simulink model "robot_lab"  (R2024b)
settings: Solver=FixedStepAuto  StartTime=0.0  StopTime=total_time  FixedStep=1e-2  RelTol=1e-3
values from neighbouring files (symbols this model uses):
  d_nom = 0.165    [MAIN_ROBOT.m]
  mode = 2    [MAIN_ROBOT.m]
  omega_L = (2*v - d_nom*w) ./ (2*r_nom)    [MAIN_ROBOT.m]
  omega_max = 10    [MAIN_ROBOT.m]
  omega_R = (2*v + d_nom*w) ./ (2*r_nom)    [MAIN_ROBOT.m]
  omega_trj = 2*pi    (= 6.28318530718)    [MAIN_ROBOT.m]
  R = 0.4    [MAIN_ROBOT.m]
  r_nom = 0.03    [MAIN_ROBOT.m]
  Ta = 1    [MAIN_ROBOT.m]
  Tc = 30    [MAIN_ROBOT.m]
  total_time = 35    [MAIN_ROBOT.m]
  Ts = 0.04    [MAIN_ROBOT.m]
undefined symbols (not defined in the file or in its folder): X, Y
libraries: robotlib x8, dspsigops x1
settings Model: SimulationMode=external  Creator=leontecosm  LastModifiedBy=leontecosm
settings OptimizationCC: DefaultParameterBehavior=Inlined  EnhancedBackFolding=on  PassReuseOutputArgsAs=Individual arguments  ZeroExternalMemoryAtStartup=off  ZeroInternalMemoryAtStartup=off  MaxStackSize=64  OptimizeBlockOrder=speed  DifferentSizesBufferReuse=on  OptimizationCustomize=off  EfficientTunableParamExpr=on
settings DebuggingCC: ParameterTunabilityLossMsg=error
settings HardwareCC: ProdBitPerPointer=32  ProdBitPerSizeT=32  ProdBitPerPtrDiffT=32  ProdLargestAtomicFloat=None  ProdIntDivRoundTo=Undefined  ProdEndianess=Unspecified  ProdWordSize=32  ProdHWDeviceType=Generic->Unspecified (assume 32-bit Generic)
settings SFSimCC: MATLABDynamicMemAlloc=off
settings RTWCC: Description=Embedded Coder  SystemTargetFile=ert.tlc  HardwareBoard=Robot Operating System (ROS)  TLCOptions="-aInlineSetEventsForThisBaseRateFcn=TLC_FALSE -aSuppressMultiTaskScheduler=TLC_FALSE  -aRateBasedStepFcn=0"  TemplateMakefile=ert_default_tmf  Toolchain=Catkin  TargetLang=C++
settings CodeAppCC: ForceParamTrailComments=on  IgnoreCustomStorageClasses=off  OperatorAnnotations=on  SimulinkDataObjDesc=on  SFDataObjDesc=on  InsertBlockDesc=on

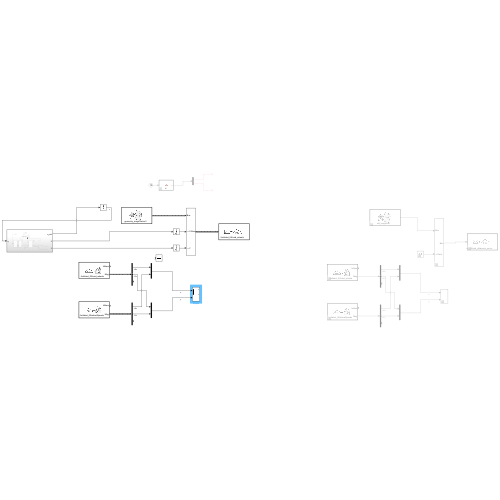
[thumbnail: Simulink's stored preview of the top-level diagram]
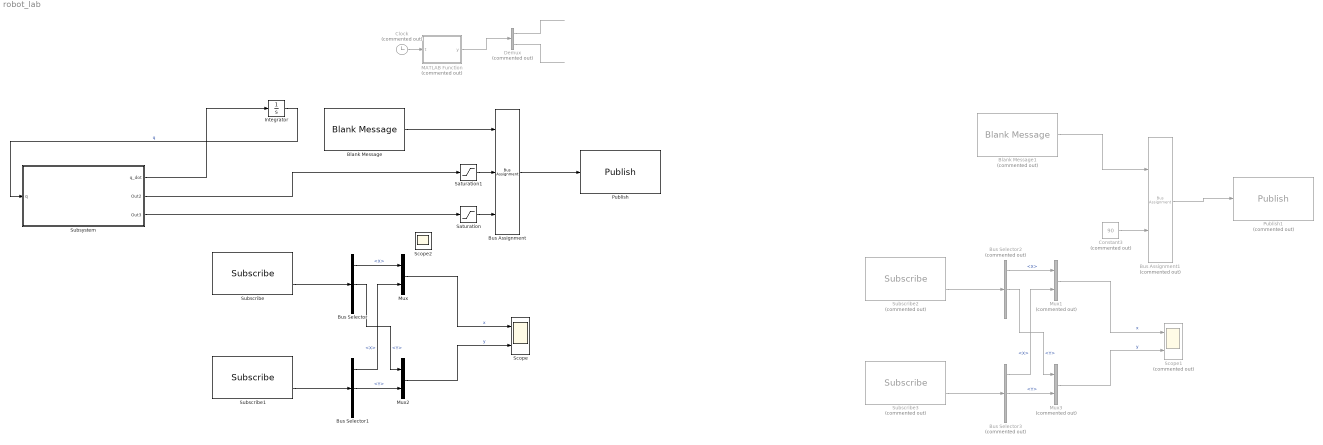
== system robot_lab ==
  Blank Message : robotlib/Blank Message  messageClass=Message  entityType=geometry_msgs/Vector3  messageType=geometry_msgs/Vector3  SampleTime=1e-2  legacyBusStruct=off
  Blank Message1 : robotlib/Blank Message  Commented=on  messageClass=Message  entityType=std_msgs/Int8  messageType=std_msgs/Int8  SampleTime=1e-1  legacyBusStruct=off
  Bus Assignment : BusAssignment  AssignedSignals=X,Y
  Bus Assignment1 : BusAssignment  Commented=on  AssignedSignals=Data
  Bus Selector : BusSelector  OutputSignals=X,Y,Z
  Bus Selector1 : BusSelector  OutputSignals=X,Y,Z
  Bus Selector2 : BusSelector  Commented=on  OutputSignals=X,Y,Z
  Bus Selector3 : BusSelector  Commented=on  OutputSignals=X,Y,Z
  Clock : Clock  Commented=on
      settings: Decimation=1/Ts
  Constant3 : Constant  Commented=on  Value=90  OutDataTypeStr=int8
  Demux : Demux  Commented=on  Outputs=2
  Integrator : Integrator  InitialCondition=[0,0,pi/3]'
  MATLAB Function : MATLAB Function  Commented=on  TreatAsAtomicUnit=on
  Mux : Mux  Inputs=2
  Mux1 : Mux  Commented=on  Inputs=2
  Mux2 : Mux  Inputs=2
  Mux3 : Mux  Commented=on  Inputs=2
  Publish : robotlib/Publish  topicSource=Select from ROS network  topic=/turtlebot_05/cmd_wheels  messageType=geometry_msgs/Vector3  legacyBusStruct=off  messageQueueLength=1
  Publish1 : robotlib/Publish  Commented=on  topicSource=Select from ROS network  topic=/turtlebot_05/cmd_ultrasonic_servo  messageType=std_msgs/Int8  legacyBusStruct=off  messageQueueLength=1
  Saturation : Saturate  UpperLimit=omega_max  LowerLimit=-omega_max
  Saturation1 : Saturate  UpperLimit=omega_max  LowerLimit=-omega_max
  Scope : Scope  NumInputPorts=2
  Scope1 : Scope  Commented=on  NumInputPorts=2
  Scope2 : Scope
  Subscribe : robotlib/Subscribe  topicSource=Select from ROS network  topic=/turtlebot_05/cmd_wheels  messageType=geometry_msgs/Vector3  SampleTime=1e-2  legacyBusStruct=off  messageQueueLength=1
  Subscribe1 : robotlib/Subscribe  topicSource=Select from ROS network  topic=/turtlebot_05/wheelSpeeds  messageType=geometry_msgs/Vector3  SampleTime=1e-2  legacyBusStruct=off  messageQueueLength=1
  Subscribe2 : robotlib/Subscribe  Commented=on  topicSource=Select from ROS network  topic=/turtlebot_05/cmd_wheels  messageType=geometry_msgs/Vector3  SampleTime=-1  legacyBusStruct=off  messageQueueLength=1
  Subscribe3 : robotlib/Subscribe  Commented=on  topicSource=Select from ROS network  topic=/turtlebot_05/wheelSpeeds  messageType=geometry_msgs/Vector3  SampleTime=-1  legacyBusStruct=off  messageQueueLength=1
  Subsystem : Subsystem
  wires:
  Blank Message/1 -> Bus Assignment/1
  Bus Assignment/1 -> Publish/1
  Saturation/1 -> Bus Assignment/3
  Saturation1/1 -> Bus Assignment/2
  Subscribe/2 -> Bus Selector/1
  Subscribe1/2 -> Bus Selector1/1
  Bus Selector/1 -> Mux/1  "<X>"
  Bus Selector1/1 -> Mux/2  "<X>"
  Bus Selector/2 -> Mux2/1  "<Y>"
  Bus Selector1/2 -> Mux2/2  "<Y>"
  Mux/1 -> Scope/1  "x"
  Mux2/1 -> Scope/2  "y"
  Mux3/1 -> Scope1/2  "y"
  Mux1/1 -> Scope1/1  "x"
  Bus Selector3/2 -> Mux3/2  "<Y>"
  Bus Selector2/2 -> Mux3/1  "<Y>"
  Bus Selector3/1 -> Mux1/2  "<X>"
  Bus Selector2/1 -> Mux1/1  "<X>"
  Subscribe3/2 -> Bus Selector3/1
  Subscribe2/2 -> Bus Selector2/1
  Constant3/1 -> Bus Assignment1/2
  Bus Assignment1/1 -> Publish1/1
  Blank Message1/1 -> Bus Assignment1/1
  Clock/1 -> MATLAB Function/1(t)
  Demux/2 -> ?
  MATLAB Function/1(y) -> Demux/1
  Demux/1 -> ?
  Integrator/1 -> Subsystem/1(q)  "q"
  Subsystem/1(q_dot) -> Integrator/1
  Subsystem/2(Out2) -> Saturation1/1
  Subsystem/3(Out3) -> Saturation/1

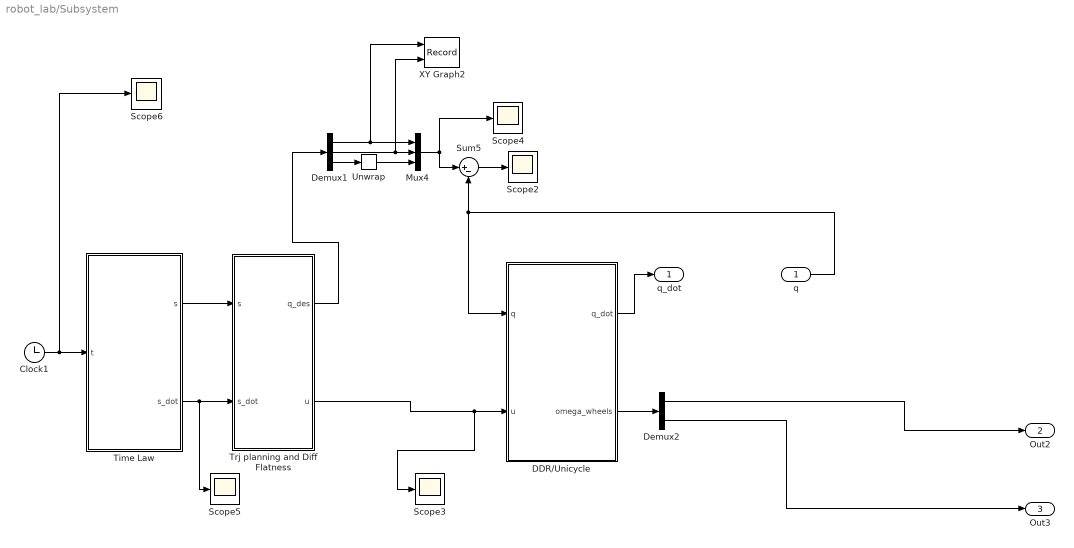
== system robot_lab/Subsystem ==
  q : Inport
  Clock1 : Clock
      settings: Decimation=1/Ts
  DDR/Unicycle : MATLAB Function  TreatAsAtomicUnit=on
  Demux1 : Demux  Outputs=3
  Demux2 : Demux  Outputs=2
  Mux4 : Mux  Inputs=3
  Scope{2..6} (5 alike) : Scope
  Sum5 : Sum  Inputs=|+-
  Time Law : MATLAB Function  TreatAsAtomicUnit=on
  Trj planning and Diff Flatness : MATLAB Function  TreatAsAtomicUnit=on
  Unwrap : dspsigops/Unwrap  tol=pi  InputProcessing=Columns as channels (frame based)  running=off
  XY Graph2 : Record  FileSettingsInternal="{\"entries\":[{\"content\":{\"excelSettings\":{\"content\":{},\"type\":\"Streamout.ExcelSettings\"}},\"type\":\"Streamout.FileSettingStorage\",\"uuid\":\"\"}],\"packageUris\":[\"http:\\/\\/schema.mathworks.com\\/mf0\\/streamout_blocks\\/R2020a\"],\"version\":\"1.0\"}"  Layout=[1 1]  SignalsInternal="{\"entries\":[{\"content\":{\"signals\":[{\"content\":{\"blockPath\":[],\"dimensions\":[1,1],\"domain\":\"\",\"lineColor\":\"#a2142f\",\"plots\":[ 1 ],\"port\":1,\"sid\":[\"\"],\"signalID\":1,\"signalName\":\"Demux1:1\"},\"type\":\"RecordBlkView.Signal\",\"uuid\":\"\"},{\"content\":{\"blockPath\":[],\"dimensions\":[1,1],\"domain\":\"\",\"lineColor\":\"#139fff\",\"plots\":[ 1 ],\"port\":2,\"sid\":[\"\"],\"signalID\":2,\"signalName\":\"Demux1:2\"},\"type\":\"RecordBlkView.Signal\",\"uuid\":\"\"}]},\"type\":\"RecordBlkView.InputSignals\",\"uuid\":\"\"}],\"packageUris\":[\"http:\\/\\/schema.mathworks.com\\/mf0\\/streamout_blocks\\/R2020a\"],\"version\":\"1.0\"}"  VisualizationBindings="{\"xyplotplugin\":{\"info\":[{\"series\":[{\"bindingParametersList\":[{\"parameter\":\"X-Axis\",\"signalID\":1,\"signalName\":\"Demux1:1\"},{\"parameter\":\"Y-Axis\",\"signalID\":2,\"signalName\":\"Demux1:2\"}],\"seriesID\":0}],\"subplotID\":1}]}}"  CompatibilityTag=XY
  q_dot : Outport
  Out2 : Outport  Port=2
  Out3 : Outport  Port=3
  wires:
  Demux1/2 -> XY Graph2/2, Mux4/2
  Demux1/1 -> XY Graph2/1, Mux4/1
  Unwrap/1 -> Mux4/3
  Trj planning and Diff Flatness/2(u) -> Scope3/1, DDR/Unicycle/2(u)
  Time Law/1(s) -> Trj planning and Diff Flatness/1(s)
  DDR/Unicycle/2(omega_wheels) -> Demux2/1
  Demux1/3 -> Unwrap/1
  Sum5/1 -> Scope2/1
  Time Law/2(s_dot) -> Scope5/1, Trj planning and Diff Flatness/2(s_dot)
  Trj planning and Diff Flatness/1(q_des) -> Demux1/1
  q/1 -> Sum5/2, DDR/Unicycle/1(q)
  Clock1/1 -> Scope6/1, Time Law/1(t)
  Mux4/1 -> Sum5/1, Scope4/1
  Demux2/2 -> Out3/1
  Demux2/1 -> Out2/1
  DDR/Unicycle/1(q_dot) -> q_dot/1

== matlab function robot_lab/Subsystem/DDR//Unicycle ==
  data: q input; u input; q_dot output; omega_wheels output; d_nom parameter; r_nom parameter
function [q_dot, omega_wheels] = DDR_Unicycle(q, u, d_nom, r_nom)
v = u(1);
omega = u(2);

q_dot = [cos(q(3))*v; sin(q(3))*v; omega];

%evaluation of speed wheels
omega_L = (2*v - d_nom*omega) / (2*r_nom);
omega_R = (2*v + d_nom*omega) / (2*r_nom);
omega_wheels=[omega_R; omega_L];

== matlab function robot_lab/MATLAB Function ==
  data: t input; y output; Ts parameter; omega_R parameter; omega_L parameter
function y = fcn(t,Ts, omega_R, omega_L)
time = t*Ts +1;

y = [omega_R(time),omega_L(time)];

== matlab function robot_lab/Subsystem/Time Law ==
  data: t input; s output; s_dot output; total_time parameter; mode parameter; Ta parameter; Tc parameter
function [s, s_dot] = fcn(t,total_time, mode,Ta, Tc)
s=0;
s_dot=0;

if mode==1%if mode =1 costasnt time law else trapezoidal
    s_dot = 1/total_time;
    s=t/total_time;
else
   

    Vc=1/(Ta+Tc);% velocità costante
    a=Vc/Ta;% acceleration
    
    switch 1 %formula on the slide
        case t<Ta
            s_dot=a*t;
            s=(a*(t^2))/2;

        case (t>=Ta)&&(t<(Tc+Ta))
            s_dot=Vc;
            s=(a*(Ta^2))/2+Vc*(t-Ta);

        case (t>=(Tc+Ta))&&(t<(Tc+2*Ta))
            s_dot=Vc-a*(t-Ta-Tc);
            s=(a*(Ta^2))/2+Vc*Tc+Vc*(t-Ta-Tc)-a*(t-Ta-Tc)^2/2;

        case t>=(Tc+2*Ta)
            s_dot=0;
            s=1;
    end

end

== matlab function robot_lab/Subsystem/Trj planning and Diff Flatness ==
  data: q_des output; u output; R parameter; omega_trj parameter; s input; s_dot input
function [q_des, u] = get_inputs(R,omega_trj, s, s_dot)

x=R*sin(2*omega_trj.*s);
y=R*sin(omega_trj.*s);

x_dot = R*2*omega_trj*cos(2*omega_trj.*s);
y_dot = R*omega_trj*cos(omega_trj.*s);

x_ddot = R*4*omega_trj*omega_trj*(-sin(2*omega_trj.*s));
y_ddot = R*omega_trj*omega_trj*(-sin(omega_trj.*s));

theta = atan2(y_dot,x_dot);

%   v
v = s_dot*sqrt(y_dot^2 + x_dot^2);

%   omega
w = s_dot*(x_dot*y_ddot - y_dot*x_ddot)/(y_dot^2 + x_dot^2);
    
q_des = [x; y; theta];
u = [v; w];
